simulink model "MdXX_QuitChk"  (R2018b)
settings: Solver=FixedStepDiscrete  StartTime=0.0  StopTime=10.0  FixedStep=0.01  RelTol=1e-3
undefined symbols (not defined in the file or in its folder): KeSMSuMdNums_Val, MdRspLocal2
libraries: simulink x1
settings Model: ModifiedHistory=2024.12.11 V3.0.0 CR955881  Creator=sn2xws  LastModifiedBy=sn55gm
settings DataIOCC: SaveFormat=StructureWithTime
settings OptimizationCC: DefaultParameterBehavior=Inlined  EnhancedBackFolding=on  PassReuseOutputArgsAs=Individual arguments  ZeroExternalMemoryAtStartup=off  ZeroInternalMemoryAtStartup=off  OptimizeBlockOrder=speed  DifferentSizesBufferReuse=on  OptimizationCustomize=off
settings DebuggingCC: ParameterTunabilityLossMsg=error
settings ModelReferenceCC: ModelReferenceNumInstancesAllowed=Single
settings SFSimCC: MATLABDynamicMemAlloc=off
settings RTWCC: SystemTargetFile=autosar.tlc  GenCodeOnly=on  TemplateMakefile=ert_default_tmf  Description=AUTOSAR  GenerateReport=on  IncludeHyperlinkInReport=on  LaunchReport=on  GenerateTraceInfo=on  GenerateTraceReport=on  GenerateTraceReportSl=on  GenerateTraceReportSf=on  GenerateTraceReportEml=on  GenerateCodeMetricsReport=on
settings CodeAppCC: ForceParamTrailComments=on  IgnoreCustomStorageClasses=off  OperatorAnnotations=on  SimulinkDataObjDesc=on  SFDataObjDesc=on  InsertBlockDesc=on
settings STFCustomTargetCC: TargetLangStandard=C99 (ISO)  MultiwordLength=256  ParMdlRefBuildCompliant=on  CompOptLevelCompliant=on  IncludeMdlTerminateFcn=off  CombineOutputUpdateFcns=on  SuppressErrorStatus=on  ERTCustomFileBanners=on  SupportNonFinite=off  SupportComplex=off  SupportContinuousTime=off  SupportNonInlinedSFcns=off  RemoveResetFunc=on  MATLABClassNameForMDSCustomization=Simulink.SoftwareTarget.ERTCustomization  AutosarCompliant=on  UseToolchainInfoCompliant=on  LookupTableObjectStructAxisOrder=2,1,3,4,...  LUTObjectStructOrderEvenSpacing=Size,Table,Breakpoints  SystemTargetFile=autosar.tlc
settings ERTTargetCC: TargetLangStandard=C99 (ISO)  ConcurrentExecutionCompliant=off  IncludeMdlTerminateFcn=off  SuppressErrorStatus=on  SupportNonFinite=off  SupportComplex=off  ModelStepFunctionPrototypeControlCompliant=off  CPPClassGenCompliant=off  AutosarCompliant=on  LookupTableObjectStructAxisOrder=2,1,3,4,...  LUTObjectStructOrderEvenSpacing=Size,Table,Breakpoints  InlinedParameterPlacement=NonHierarchical  ERTCustomFileTemplate=example_file_process.tlc  ERTFilePackagingFormat=Compact

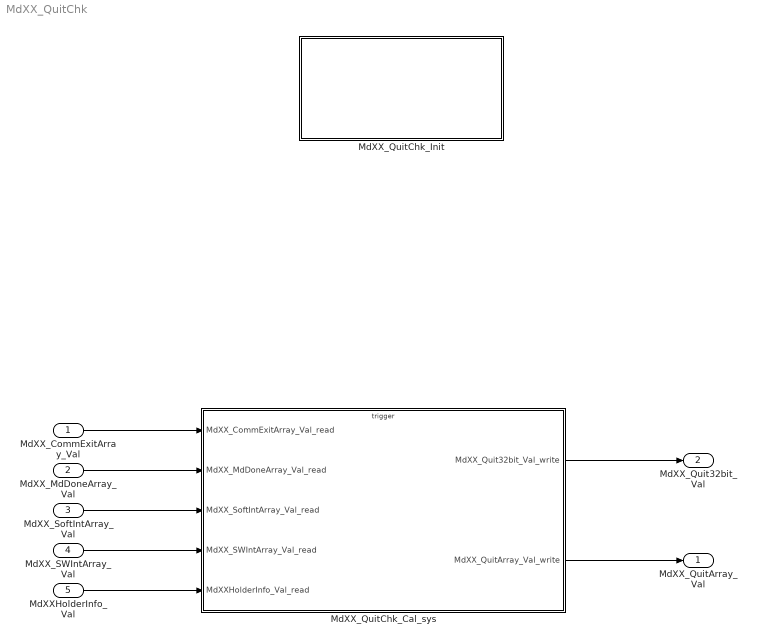
== system MdXX_QuitChk ==
  MdXX_CommExitArray_Val : Inport  OutDataTypeStr=boolean  PortDimensions=32
  MdXX_MdDoneArray_Val : Inport  Port=2  OutDataTypeStr=uint8  PortDimensions=32
  MdXX_SoftIntArray_Val : Inport  Port=3  OutDataTypeStr=boolean  PortDimensions=32
  MdXX_SWIntArray_Val : Inport  Port=4  OutDataTypeStr=boolean  PortDimensions=32
  MdXXHolderInfo_Val : Inport  Port=5  OutDataTypeStr=uint32  PortDimensions=1
  MdXX_QuitChk_Cal_sys : Subsystem
  MdXX_QuitChk_Init : Subsystem
  MdXX_QuitArray_Val : Outport  OutDataTypeStr=Enum: MdRspLocal2  PortDimensions=32
  MdXX_Quit32bit_Val : Outport  Port=2  OutDataTypeStr=uint32  PortDimensions=1
  wires:
  MdXX_CommExitArray_Val/1 -> MdXX_QuitChk_Cal_sys/1(MdXX_CommExitArray_Val_read)
  MdXX_MdDoneArray_Val/1 -> MdXX_QuitChk_Cal_sys/2(MdXX_MdDoneArray_Val_read)
  MdXX_SoftIntArray_Val/1 -> MdXX_QuitChk_Cal_sys/3(MdXX_SoftIntArray_Val_read)
  MdXX_SWIntArray_Val/1 -> MdXX_QuitChk_Cal_sys/4(MdXX_SWIntArray_Val_read)
  MdXX_QuitChk_Cal_sys/2(MdXX_QuitArray_Val_write) -> MdXX_QuitArray_Val/1
  MdXX_QuitChk_Cal_sys/1(MdXX_Quit32bit_Val_write) -> MdXX_Quit32bit_Val/1
  MdXXHolderInfo_Val/1 -> MdXX_QuitChk_Cal_sys/5(MdXXHolderInfo_Val_read)

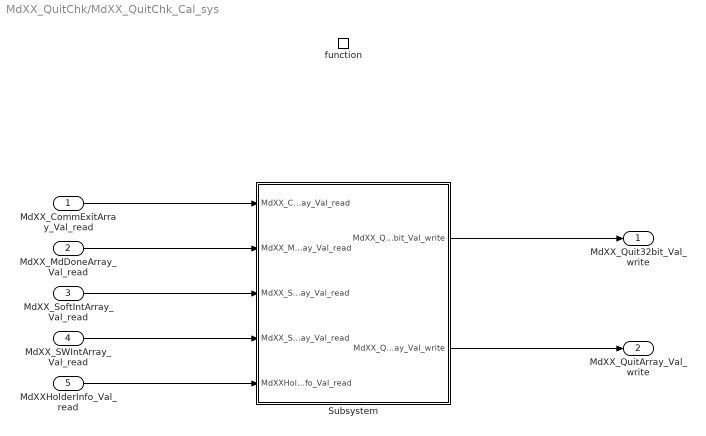
== system MdXX_QuitChk/MdXX_QuitChk_Cal_sys ==
  MdXX_CommExitArray_Val_read : Inport
  MdXX_MdDoneArray_Val_read : Inport  Port=2
  MdXX_SoftIntArray_Val_read : Inport  Port=3
  MdXX_SWIntArray_Val_read : Inport  Port=4
  MdXXHolderInfo_Val_read : Inport  Port=5
  function : TriggerPort  TriggerType=function-call  IsSimulinkFunction=on  FunctionName=MdXX_QuitChk_Cal  VariantControl=(inherit)
  Subsystem : Subsystem
  MdXX_Quit32bit_Val_write : Outport
  MdXX_QuitArray_Val_write : Outport  Port=2
  wires:
  MdXX_CommExitArray_Val_read/1 -> Subsystem/1(MdXX_CommExitArray_Val_read)
  MdXX_MdDoneArray_Val_read/1 -> Subsystem/2(MdXX_MdDoneArray_Val_read)
  MdXX_SoftIntArray_Val_read/1 -> Subsystem/3(MdXX_SoftIntArray_Val_read)
  MdXX_SWIntArray_Val_read/1 -> Subsystem/4(MdXX_SWIntArray_Val_read)
  Subsystem/1(MdXX_Quit32bit_Val_write) -> MdXX_Quit32bit_Val_write/1
  Subsystem/2(MdXX_QuitArray_Val_write) -> MdXX_QuitArray_Val_write/1
  MdXXHolderInfo_Val_read/1 -> Subsystem/5(MdXXHolderInfo_Val_read)

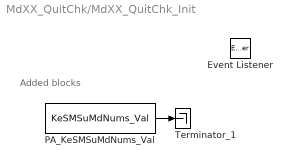
== system MdXX_QuitChk/MdXX_QuitChk_Init ==
  note: Added blocks
  Event Listener : EventListener  EventName=reset
  PA_KeSMSuMdNums_Val : Constant  Value=KeSMSuMdNums_Val
  Terminator_1 : Terminator
  wires:
  PA_KeSMSuMdNums_Val/1 -> Terminator_1/1

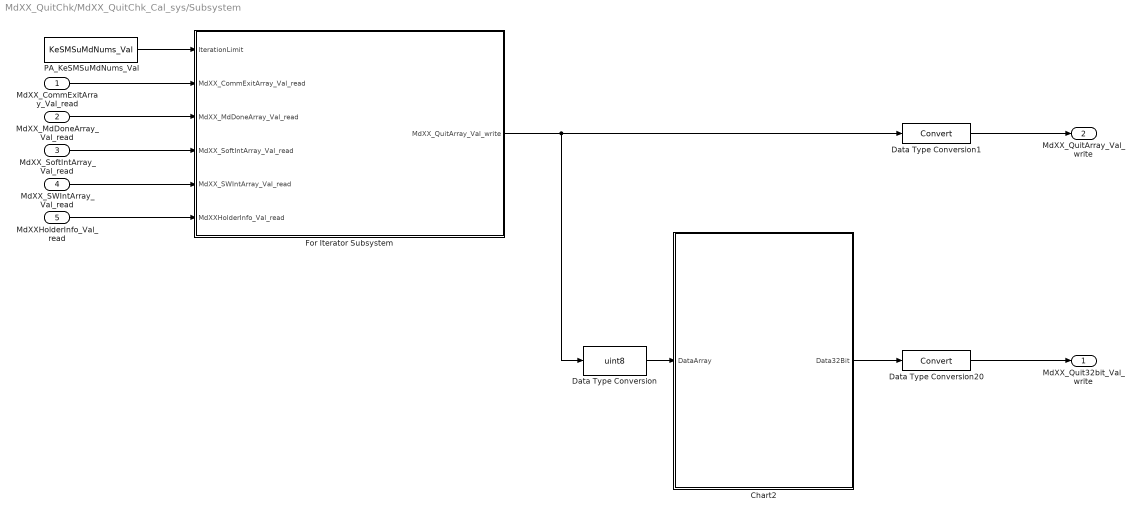
== system MdXX_QuitChk/MdXX_QuitChk_Cal_sys/Subsystem ==
  MdXX_CommExitArray_Val_read : Inport
  MdXX_MdDoneArray_Val_read : Inport  Port=2
  MdXX_SoftIntArray_Val_read : Inport  Port=3
  MdXX_SWIntArray_Val_read : Inport  Port=4
  MdXXHolderInfo_Val_read : Inport  Port=5
  Chart2 : Stateflow chart  TreatAsAtomicUnit=on
  Data Type Conversion : DataTypeConversion  OutDataTypeStr=uint8
  Data Type Conversion1 : DataTypeConversion
  Data Type Conversion20 : DataTypeConversion
  For Iterator Subsystem : Subsystem  TreatAsAtomicUnit=on
  PA_KeSMSuMdNums_Val : Constant  Value=KeSMSuMdNums_Val
  MdXX_Quit32bit_Val_write : Outport
  MdXX_QuitArray_Val_write : Outport  Port=2
  wires:
  PA_KeSMSuMdNums_Val/1 -> For Iterator Subsystem/1(IterationLimit)
  Data Type Conversion20/1 -> MdXX_Quit32bit_Val_write/1
  MdXX_CommExitArray_Val_read/1 -> For Iterator Subsystem/2(MdXX_CommExitArray_Val_read)
  MdXX_MdDoneArray_Val_read/1 -> For Iterator Subsystem/3(MdXX_MdDoneArray_Val_read)
  MdXX_SoftIntArray_Val_read/1 -> For Iterator Subsystem/4(MdXX_SoftIntArray_Val_read)
  MdXX_SWIntArray_Val_read/1 -> For Iterator Subsystem/5(MdXX_SWIntArray_Val_read)
  For Iterator Subsystem/1(MdXX_QuitArray_Val_write) -> Data Type Conversion/1, Data Type Conversion1/1
  Chart2/1(Data32Bit) -> Data Type Conversion20/1
  Data Type Conversion/1 -> Chart2/1(DataArray)
  Data Type Conversion1/1 -> MdXX_QuitArray_Val_write/1
  MdXXHolderInfo_Val_read/1 -> For Iterator Subsystem/6(MdXXHolderInfo_Val_read)

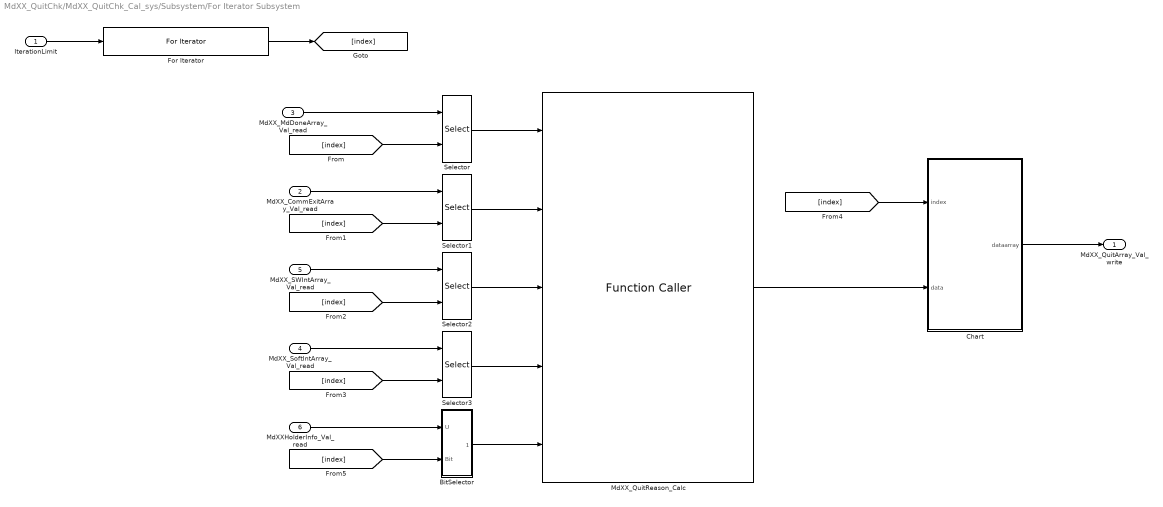
== system MdXX_QuitChk/MdXX_QuitChk_Cal_sys/Subsystem/For Iterator Subsystem ==
  IterationLimit : Inport
  MdXX_CommExitArray_Val_read : Inport  Port=2
  MdXX_MdDoneArray_Val_read : Inport  Port=3
  MdXX_SoftIntArray_Val_read : Inport  Port=4
  MdXX_SWIntArray_Val_read : Inport  Port=5
  MdXXHolderInfo_Val_read : Inport  Port=6
  BitSelector : Subsystem
  Chart : Stateflow chart  TreatAsAtomicUnit=on
  For Iterator : ForIterator  IterationSource=external  IndexMode=Zero-based  IterationVariableDataType=int8
  MdXX_QuitReason_Calc : FunctionCaller  FunctionPrototype=MdQuitReason = MdXX_QuitReason_Calc(MdDone,ExitCond,SWInt,SoftInt,MdHoldInfo)  InputArgumentSpecifications=uint8(1), boolean(true), boolean(true), boolean(true), boolean(true)  OutputArgumentSpecifications=MdRspLocal2(0)
  Selector{,1..3} (4 alike) : Selector  IndexMode=Zero-based  InputPortWidth=32  IndexOptions=Index vector (port)  Indices=[1 3]  OutputSizes=1
  MdXX_QuitArray_Val_write : Outport
  wires:
  IterationLimit/1 -> For Iterator/1
  MdXX_SWIntArray_Val_read/1 -> Selector2/1
  MdXX_MdDoneArray_Val_read/1 -> Selector/1
  MdXX_CommExitArray_Val_read/1 -> Selector1/1
  For Iterator/1 -> [index]
  [index] -> Selector/2
  Selector/1 -> MdXX_QuitReason_Calc/1
  Selector1/1 -> MdXX_QuitReason_Calc/2
  Selector2/1 -> MdXX_QuitReason_Calc/3
  Selector3/1 -> MdXX_QuitReason_Calc/4
  [index] -> Selector1/2
  [index] -> Selector2/2
  [index] -> Selector3/2
  MdXX_SoftIntArray_Val_read/1 -> Selector3/1
  MdXX_QuitReason_Calc/1 -> Chart/2(data)
  Chart/1(dataarray) -> MdXX_QuitArray_Val_write/1
  [index] -> Chart/1(index)
  BitSelector/1(BitOut) -> MdXX_QuitReason_Calc/5
  MdXXHolderInfo_Val_read/1 -> BitSelector/1(U)
  [index] -> BitSelector/2(Bit)

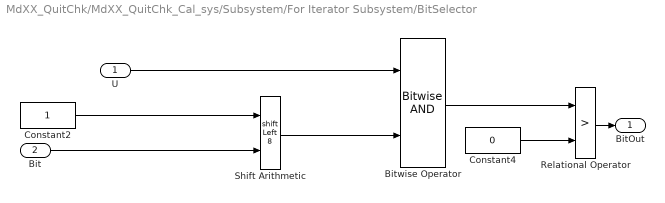
== system MdXX_QuitChk/MdXX_QuitChk_Cal_sys/Subsystem/For Iterator Subsystem/BitSelector ==
  U : Inport
  Bit : Inport  Port=2
  Bitwise Operator : simulink/Logic and Bit Operations/Bitwise Operator  logicop=AND  UseBitMask=off  NumInputPorts=2  BitMask=bin2dec('11011001')  BitMaskRealWorld=Stored Integer
  Constant2 : Constant  OutDataTypeStr=uint32
  Constant4 : Constant  Value=0  OutDataTypeStr=uint32
  Relational Operator : RelationalOperator  Operator=>  OutDataTypeStr=boolean  RndMeth=Simplest
  Shift Arithmetic : ArithShift  BitShiftNumberSource=Input port  BitShiftNumber=8  BitShiftDirection=Left
      settings: InputPortMap=u0,p1
  BitOut : Outport
  wires:
  Relational Operator/1 -> BitOut/1
  Constant4/1 -> Relational Operator/2
  Constant2/1 -> Shift Arithmetic/1
  Bitwise Operator/1 -> Relational Operator/1
  U/1 -> Bitwise Operator/1
  Shift Arithmetic/1 -> Bitwise Operator/2
  Bit/1 -> Shift Arithmetic/2

== stateflow chart MdXX_QuitChk/MdXX_QuitChk_Cal_sys/Subsystem/Chart2 ==
  (default) -> (junction 3) : {Data32Bit = 0x00000000;}
  (junction 3) -> (junction 9) : {i = 0;}
  (junction 9) -> (junction 4) [order 1] : [i < 32]
  (junction 4) -> (junction 1) : {
      | temp_var = uint32(DataArray[i]!=0);
      | temp_var= temp_var << i;
      | Data32Bit = Data32Bit |  temp_var;
      | }
  (junction 1) -> (junction 9) : {i++;}
  (junction 9) -> (junction 5) [order 2]
  data: Data32Bit output uint32; DataArray input uint8 size=32; temp_var local uint32; i local uint8

== stateflow chart MdXX_QuitChk/MdXX_QuitChk_Cal_sys/Subsystem/For Iterator Subsystem/Chart ==
  (default) -> (junction 1)
  (junction 1) -> (junction 6) : {
      | dataarray[index]=data;
      | }
  data: index input int8; data input Enum: MdRspLocal2; dataarray output Enum: MdRspLocal2 size=32
